simulink model "sim_linear_control_psi"  (R2018a)
settings: Solver=ode3  StartTime=0.0  StopTime=5  FixedStep=0.001  RelTol=1e-3
values from neighbouring files (symbols this model uses):
  CA = C*A    [lin_control_error.m]    (also in lin_control_psi.m; lin_control_y.m)
  invCB = pinv(C*B)    [lin_control_error.m]    (also in lin_control_psi.m; lin_control_y.m)
  Kb_psi = 1    [lin_control_psi.m]
  Kb_r = 4    [lin_control_psi.m]
  Vx = 30    [lin_control_error.m]    (also in lin_control_psi.m = 8.33333333333; lin_control_y.m = 8.33333333333)
settings Model: Creator=E183308  LastModifiedBy=E183308

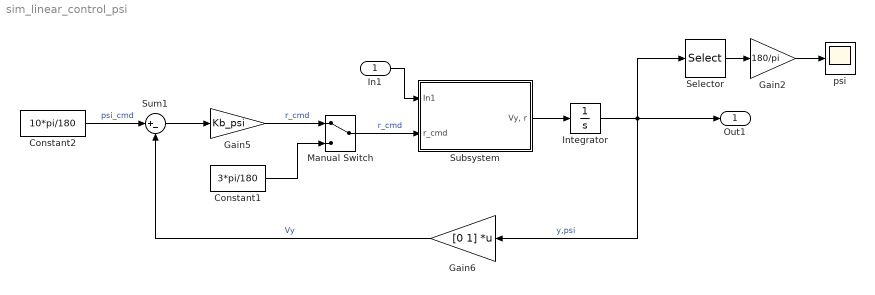
== system sim_linear_control_psi ==
  In1 : Inport
  Constant1 : Constant  Value=3*pi/180
  Constant2 : Constant  Value=10*pi/180
  Gain2 : Gain  Gain=180/pi
  Gain5 : Gain  Gain=Kb_psi
  Gain6 : Gain  Gain=[0 1]  Multiplication=Matrix(K*u)
  Integrator : Integrator
  Manual Switch : ManualSwitch
  Selector : Selector  InputPortWidth=2  IndexOptions=Index vector (dialog)  Indices=2  OutputSizes=1
  Subsystem : Subsystem
  Sum1 : Sum  Inputs=|+-
  psi : Scope
  Out1 : Outport
  wires:
  Constant1/1 -> Manual Switch/2
  Constant2/1 -> Sum1/1  "psi_cmd"
  Gain5/1 -> Manual Switch/1  "r_cmd"
  Sum1/1 -> Gain5/1
  Gain6/1 -> Sum1/2  "Vy"
  Subsystem/1("Vy, r") -> Integrator/1
  In1/1 -> Subsystem/1(In1)
  Manual Switch/1 -> Subsystem/2(r_cmd)  "r_cmd"
  Integrator/1 -> Selector/1, Out1/1, Gain6/1  "y,psi"
  Gain2/1 -> psi/1
  Selector/1 -> Gain2/1

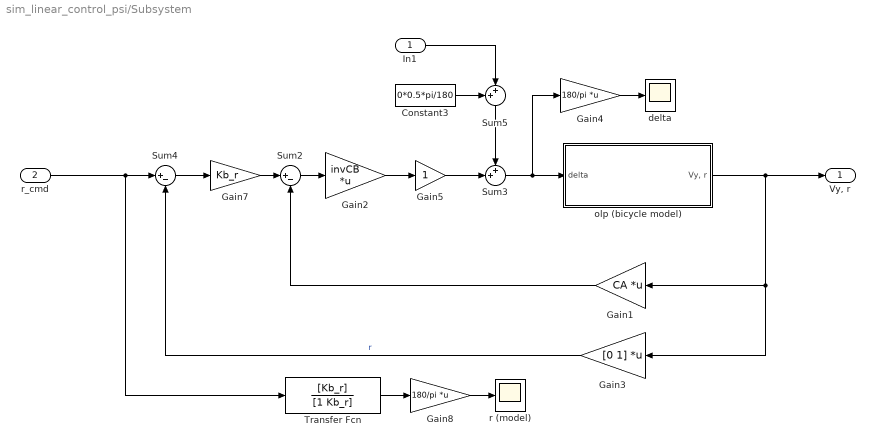
== system sim_linear_control_psi/Subsystem ==
  In1 : Inport
  r_cmd : Inport  Port=2
  Constant3 : Constant  Value=0*0.5*pi/180
  Gain1 : Gain  Gain=CA  Multiplication=Matrix(K*u)
  Gain2 : Gain  Gain=invCB  Multiplication=Matrix(K*u)
  Gain3 : Gain  Gain=[0 1]  Multiplication=Matrix(K*u)
  Gain4 : Gain  Gain=180/pi  Multiplication=Matrix(K*u)
  Gain5 : Gain
  Gain7 : Gain  Gain=Kb_r
  Gain8 : Gain  Gain=180/pi  Multiplication=Matrix(K*u)
  Sum2 : Sum  Inputs=|+-
  Sum3 : Sum  Inputs=++|
  Sum4 : Sum  Inputs=|+-
  Sum5 : Sum  Inputs=++|
  Transfer Fcn : TransferFcn  Numerator=[Kb_r]  Denominator=[1 Kb_r]
  delta : Scope
  olp (bicycle model) : Subsystem
  r (model) : Scope
  "Vy, r" : Outport
  wires:
  Gain4/1 -> delta/1
  r_cmd/1 -> Transfer Fcn/1, Sum4/1
  Gain3/1 -> Sum4/2  "r"
  Transfer Fcn/1 -> Gain8/1
  Gain8/1 -> r (model)/1
  Gain2/1 -> Gain5/1
  Sum2/1 -> Gain2/1
  Sum3/1 -> Gain4/1, olp (bicycle model)/1(delta)
  Sum4/1 -> Gain7/1
  Constant3/1 -> Sum5/1
  Sum5/1 -> Sum3/1
  Gain1/1 -> Sum2/2
  Gain7/1 -> Sum2/1
  In1/1 -> Sum5/2
  olp (bicycle model)/1("Vy, r") -> Gain3/1, Gain1/1, "Vy, r"/1
  Gain5/1 -> Sum3/2

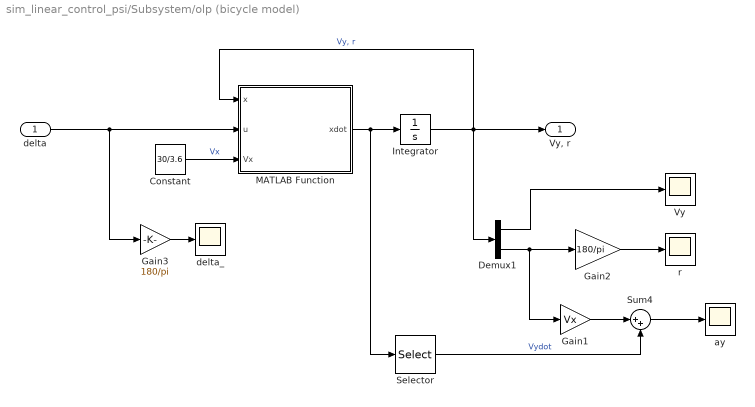
== system sim_linear_control_psi/Subsystem/olp (bicycle model) ==
  delta : Inport
  Constant : Constant  Value=30/3.6
  Demux1 : Demux  Outputs=2
  Gain1 : Gain  Gain=Vx
  Gain2 : Gain  Gain=180/pi
  Gain3 : Gain  Gain=180/pi
  Integrator : Integrator  InitialCondition=[0;0]
  MATLAB Function : MATLAB Function  TreatAsAtomicUnit=on
  Selector : Selector  InputPortWidth=2  IndexOptions=Index vector (dialog)  Indices=1  OutputSizes=1
  Sum4 : Sum  Inputs=|++
  Vy : Scope
  ay : Scope
  delta_ : Scope
  r : Scope
  "Vy, r" : Outport
  wires:
  Gain2/1 -> r/1
  Demux1/2 -> Gain1/1, Gain2/1
  Integrator/1 -> MATLAB Function/1(x), "Vy, r"/1, Demux1/1  "Vy, r"
  Gain3/1 -> delta_/1
  delta/1 -> Gain3/1, MATLAB Function/2(u)
  Constant/1 -> MATLAB Function/3(Vx)  "Vx"
  MATLAB Function/1(xdot) -> Selector/1, Integrator/1
  Demux1/1 -> Vy/1
  Gain1/1 -> Sum4/1
  Selector/1 -> Sum4/2  "Vydot"
  Sum4/1 -> ay/1

== matlab function sim_linear_control_psi/Subsystem/olp (bicycle model)/MATLAB Function ==
  data: x input; u input; xdot output; Vx input
function xdot = dynamic_lin(x,u,Vx)

% sports sedan

m = 1724; % kg
Iz = 3400; % kg/m^2
a = 1.35; % m
b = 1.15; % m
Cf = 12*1e4; % N/rad
Cr = 175*1e3; % N/rad
mu = 0.5225;

% x = [vy r]
% u = delta

A = [-(Cf+Cr)/(m*Vx)  -(a*Cf-b*Cr)/(m*Vx)-Vx; 
    -(a*Cf-b*Cr)/(Iz*Vx) -(a^2*Cf+b^2*Cr)/(Iz*Vx)];

B = [Cf/m; a*Cf/Iz];

xdot = A*x + B*u;
